simulink model "dwa"  (R2022b)
settings: Solver=VariableStepAuto  StartTime=0.0  StopTime=10  MaxStep=0.01  RelTol=1e-3
libraries: simulink x1
settings Model: Creator=zuzanna  LastModifiedBy=zuzanna

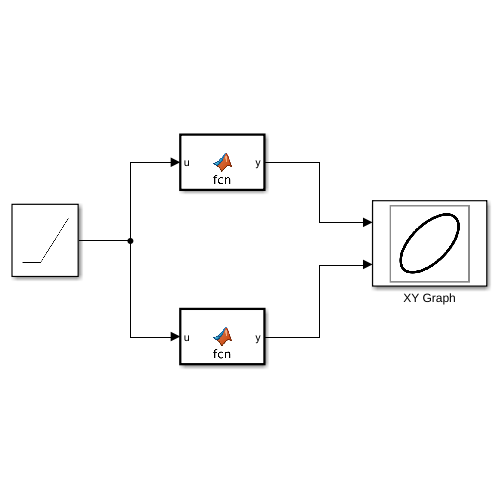
[thumbnail: Simulink's stored preview of the top-level diagram]
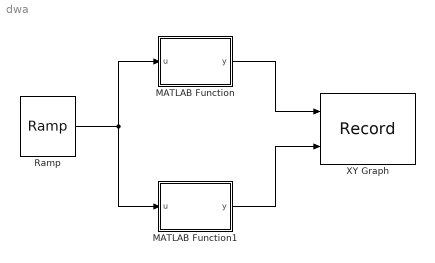
== system dwa ==
  MATLAB Function : MATLAB Function  TreatAsAtomicUnit=on
  MATLAB Function1 : MATLAB Function  TreatAsAtomicUnit=on
  Ramp : simulink/Sources/Ramp  slope=1  start=0  InitialOutput=0
  XY Graph : Record  RecordToWorkspace=on  FileSettingsInternal="{\"entries\":[{\"content\":{\"excelSettings\":{\"content\":{},\"type\":\"Streamout.ExcelSettings\"}},\"type\":\"Streamout.FileSettingStorage\",\"uuid\":\"b76e6d8c-35ad-420e-9900-64205c36551e\"}],\"packageUris\":[\"http://schema.mathworks.com/mf0/streamout_blocks/R2020a\"],\"version\":\"1.0\"}"  Layout=[1 1]  SignalsInternal="{\"entries\":[{\"content\":{\"signals\":[{\"content\":{\"blockPath\":[\"dwa/XY Graph\"],\"channel\":[],\"dimensions\":[1],\"domain\":\"dwa/XY Graph\",\"lineColor\":\"#77ac30\",\"plots\":[],\"port\":1,\"sid\":[\"\"],\"signalID\":122,\"signalName\":\"MATLAB Function\"},\"type\":\"RecordBlkView.Signal\",\"uuid\":\"6a148c6e-a2be-4236-95a0-86d77d006ee3\"},{\"content\":{\"blockPath\":[\"dwa/XY Graph\"],\"channel\":[],\"dimensions\":[1],\"domain\":\"dwa/XY Graph\",\"lineColor\":\"#4dbeee\",\"plots\":[],\"port\":2,\"sid\":[\"\"],\"signalID\":126,\"signalName\":\"MATLAB Function1\"},\"type\":\"RecordBlkView.Signal\",\"uuid\":\"182c201d-6d5d-4d94-b74e-23536f7a2883\"}]},\"type\":\"RecordBlkView.InputSignals\",\"uuid\":\"0b4a5b59-61ae-411a-bfec-651fe1bbb3f2\"}],\"packageUris\":[\"http://schema.mathworks.com/mf0/streamout_blocks/R2020a\"],\"version\":\"1.0\"}"  VisualizationBindings="{\"xyplotplugin\":{\"info\":[{\"series\":[],\"subplotID\":1}]}}"  CompatibilityTag=XY
  wires:
  Ramp/1 -> MATLAB Function1/1(u), MATLAB Function/1(u)
  MATLAB Function/1(y) -> XY Graph/1
  MATLAB Function1/1(y) -> XY Graph/2

== matlab function dwa/MATLAB Function ==
  data: u input; y output
function y = fcn(u)

y = 1/(1+u*u);

== matlab function dwa/MATLAB Function1 ==
  data: u input; y output
function y = fcn(u)

y = -u/(1+u*u);
